simulink model "Architecture_1p0"  (R2024b)
settings: Solver=VariableStepAuto  StartTime=0.0  StopTime=10.0  RelTol=1e-3
settings Model: Creator=account  LastModifiedBy=kara.28

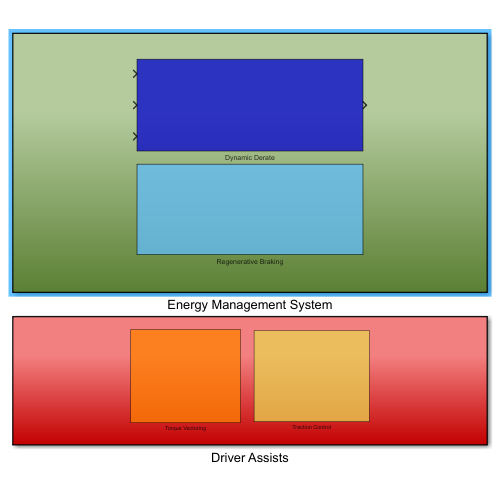
[thumbnail: Simulink's stored preview of the top-level diagram]
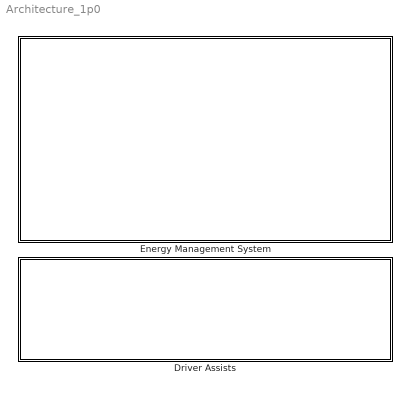
== system Architecture_1p0 ==
  Driver Assists : Subsystem
  Energy Management System : Subsystem

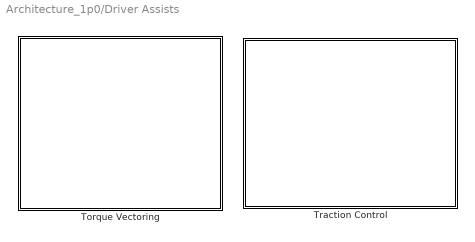
== system Architecture_1p0/Driver Assists ==
  Torque Vectoring : Subsystem
  Traction Control : Subsystem

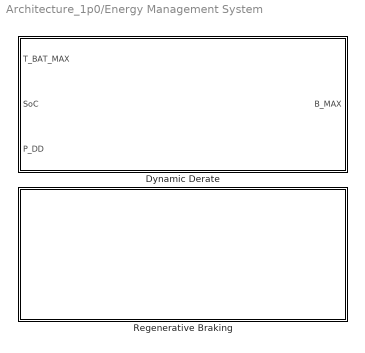
== system Architecture_1p0/Energy Management System ==
  Dynamic Derate : Subsystem
  Regenerative Braking : Subsystem

== system Architecture_1p0/Driver Assists/Torque Vectoring ==

== system Architecture_1p0/Driver Assists/Traction Control ==

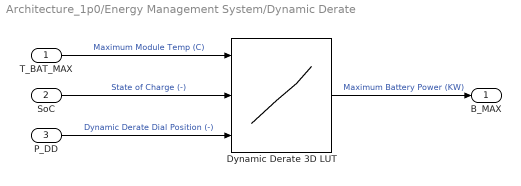
== system Architecture_1p0/Energy Management System/Dynamic Derate ==
  T_BAT_MAX : Inport
  SoC : Inport  Port=2
  P_DD : Inport  Port=3
  Dynamic Derate 3D LUT : Lookup_n-D  NumberOfTableDimensions=3  BreakpointsForDimension3=[5, 7]  Table=reshape(repmat([4 5 6;16 19 20;10 18 23],1,2),[3,3,2])  InternalRulePriority=Speed  RndMeth=Simplest
      settings: InputPortMap=u0,u1,u2
  B_MAX : Outport
  wires:
  T_BAT_MAX/1 -> Dynamic Derate 3D LUT/1  "Maximum Module Temp (C)"
  SoC/1 -> Dynamic Derate 3D LUT/2  "State of Charge (-)"
  P_DD/1 -> Dynamic Derate 3D LUT/3  "Dynamic Derate Dial Position (-)"
  Dynamic Derate 3D LUT/1 -> B_MAX/1  "Maximum Battery Power (KW)"

== system Architecture_1p0/Energy Management System/Regenerative Braking ==
